simulink model "Anti_Windup_Simu_2015"  (Simulink 8.6)
settings: Solver=FixedStepAuto  SolverMode=SingleTasking  StartTime=0.0  StopTime=100  FixedStep=0.05  RelTol=1e-3
undefined symbols (not defined in the file): Kp, ti, tw, umax, umin
libraries: cstblocks x2
settings Model: Creator=Sergio  LastModifiedBy=Sergio
settings DataIOCC: LimitDataPoints=off  SaveFormat=Dataset  SignalLoggingSaveFormat=Dataset  ReturnWorkspaceOutputs=on
settings OptimizationCC: ExpressionDepthLimit=128
settings DebuggingCC: UnderspecifiedInitializationDetection=Simplified  MergeDetectMultiDrivingBlocksExec=error  SolverPrmCheckMsg=none  FcnCallInpInsideContextMsg=EnableAllAsError  AllowSymbolicDim=on  StateNameClashWarn=none  SFUnexpectedBacktrackingDiag=error  SFNoUnconditionalDefaultTransitionDiag=error
settings HardwareCC: ProdBitPerPointer=64  ProdLargestAtomicFloat=Float  ProdIntDivRoundTo=Zero  ProdEndianess=LittleEndian  ProdWordSize=64  ProdHWDeviceType=Intel->x86-64 (Windows64)
settings ModelReferenceCC: PropagateSignalLabelsOutOfModel=on
settings SFSimCC: SimUseLocalCustomCode=on
settings RTWCC: RTWUseLocalCustomCode=on
settings GRTTargetCC: TargetLangStandard=C99 (ISO)  CombineOutputUpdateFcns=on  GRTInterface=off
settings ConfigComp: CovMetricSettings=dwe  CovHtmlReporting=off  CovSaveCumulativeToWorkspaceVar=off  CovSaveSingleToWorkspaceVar=off  CovExternalEMLEnable=on

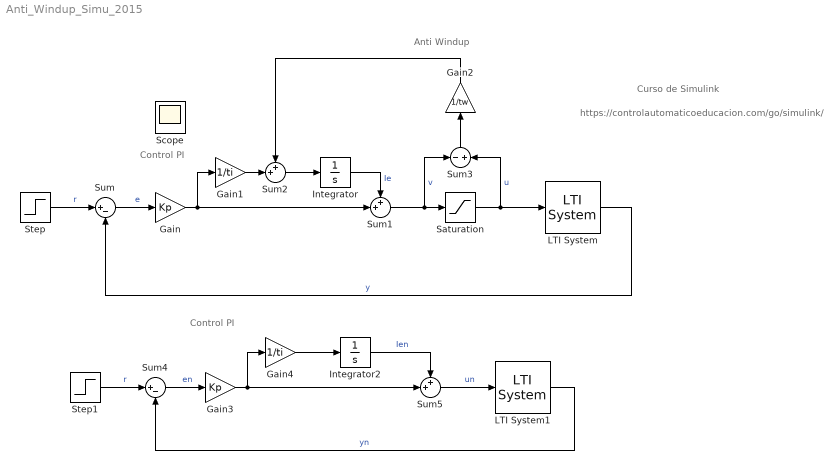
== system Anti_Windup_Simu_2015 ==
  note: https://controlautomaticoeducacion.com/go/simulink/
  note: Curso de Simulink
  note: Anti Windup
  note: Control PI
  note: Control PI
  Gain : Gain  Gain=Kp
  Gain1 : Gain  Gain=1/ti
  Gain2 : Gain  Gain=1/tw
  Gain3 : Gain  Gain=Kp
  Gain4 : Gain  Gain=1/ti
  Integrator : Integrator
  Integrator2 : Integrator
  LTI System : cstblocks/LTI System  sys=G  IC=[]
  LTI System1 : cstblocks/LTI System  sys=G  IC=[]
  Saturation : Saturate  UpperLimit=umax  LowerLimit=umin
  Step : Step  Time=10  After=0.5  SampleTime=0
  Step1 : Step  Time=10  After=0.5  SampleTime=0
  Sum : Sum  Inputs=|+-
  Sum1 : Sum  Inputs=++|
  Sum2 : Sum  Inputs=++|
  Sum3 : Sum  Inputs=-|+
  Sum4 : Sum  Inputs=|+-
  Sum5 : Sum  Inputs=++|
  Scope : Scope
  wires:
  Step/1 -> Sum/1  "r"
  LTI System/1 -> Sum/2  "y"
  Saturation/1 -> Sum3/2, LTI System/1  "u"
  Sum/1 -> Gain/1  "e"
  Gain/1 -> Sum1/2, Gain1/1
  Sum2/1 -> Integrator/1
  Sum1/1 -> Sum3/1, Saturation/1  "v"
  Sum3/1 -> Gain2/1
  Gain1/1 -> Sum2/2
  Gain2/1 -> Sum2/1
  Integrator/1 -> Sum1/1  "Ie"
  Integrator2/1 -> Sum5/1  "Ien"
  Sum5/1 -> LTI System1/1  "un"
  Gain4/1 -> Integrator2/1
  Gain3/1 -> Gain4/1, Sum5/2
  Sum4/1 -> Gain3/1  "en"
  LTI System1/1 -> Sum4/2  "yn"
  Step1/1 -> Sum4/1  "r"
